simulink model "Vicon_16Aug2012"  (Simulink 7.7)
settings: Solver=ode4  StartTime=0.0  StopTime=inf  FixedStep=sample_time  RelTol=1e-3
InitFcn:
  | sample_time=0.02;
undefined symbols (not defined in the file or in its folder): DiscIntNeverNeededParam
libraries: simulink x7, utility x1
(part 1 of 2)
settings Model: Creator=ttcl3  LastModifiedBy=Zhao Weihua
settings SolverCC: MaxConsecutiveMinStep=auto
settings DebuggingCC: MultiTaskRateTransMsg=warning

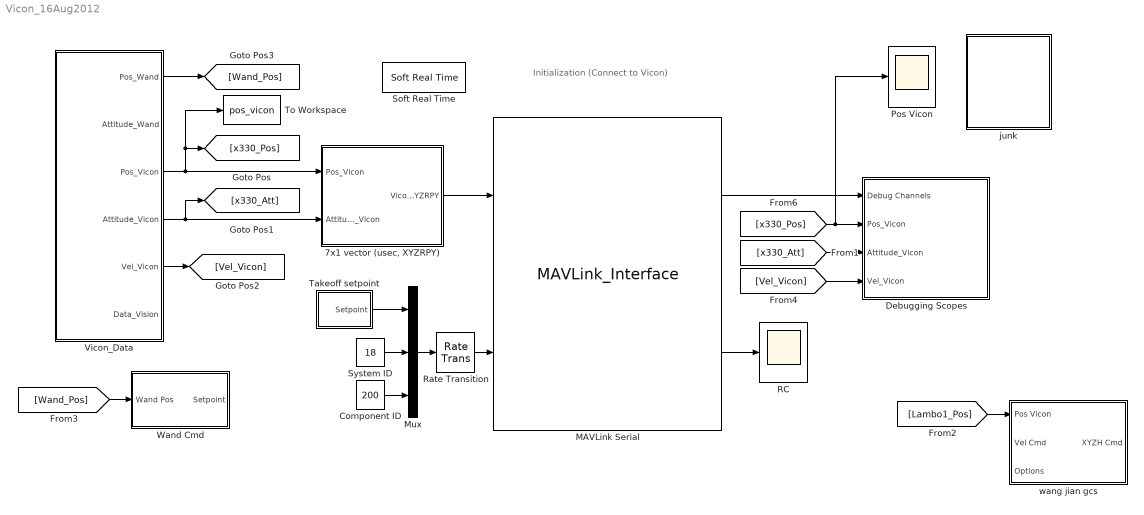
== system Vicon_16Aug2012 ==
  note: Initialization
      | (Connect to Vicon)
  "7x1 vector (usec, XYZRPY)" : Subsystem
  Component ID : Constant  Value=200  SampleTime=sample_time
  Debugging Scopes : Subsystem
  MAVLink Serial : S-Function  FunctionName=MAVLink_Interface  Parameters=COM_Port,Baud_Rate,MSG_INPUT,MSG_OUTPUT  EnableBusSupport=off  mask{COM_Port='COM8', Baud_Rate=57600, HEART_BEAT=off, ATTITUDE_OUT=on, RAW_IMU=off, POSITION_OUT=off, VFR_HUD=off, RC_SCALED=on, SERVO_OUT_RAW=off, VICON_XYZ_RPY_Output=off, SET_MODE=off, DATA_STREAM=off, ATTITUDE_COMMAND=off, ATTITUDE_IN=off, GPS_RAW_IN=off, VFR_HUD_IN=off, VICON_XYZ_RPY=on, VICON_VEL=off, POSITION_DESIRED=on}
      mask prompts: COM_Port "COM Port"; Baud_Rate "Baud Rate"; HEART_BEAT "HEART BEAT"; ATTITUDE_OUT "ATTITUDE"; RAW_IMU "RAW IMU"; POSITION_OUT "GLOBAL POSITION"; VFR_HUD "VFR HUD"; RC_SCALED "RC CHANNELS SCALED"; SERVO_OUT_RAW "SERVO OUTPUT RAW"; VICON_XYZ_RPY_Output "VICON Output"; SET_MODE "SET MODE"; DATA_STREAM "REQUEST DATA STREAM"; ATTITUDE_COMMAND "ATTITUDE COMMAND"; ATTITUDE_IN "ATTITUDE (HIL)"; GPS_RAW_IN "GPS RAW (HIL)"; VFR_HUD_IN "AIRSPEED (HIL)"; VICON_XYZ_RPY "VICON POSITION"; VICON_VEL "VICON SPEED"; POSITION_DESIRED "Position Desired"
      mask init:
      | MSG_ID_NUM_INPUT = [uint8(11) uint8(66) uint8(59) uint8(30) uint8(32) uint8(73) uint8(104) uint8(103) uint8(50)];
      | MSG_ID_NAME_INPUT = [SET_MODE DATA_STREAM ATTITUDE_COMMAND ATTITUDE_IN GPS_RAW_IN VFR_HUD_IN VICON_XYZ_RPY VICON_VEL POSITION_DESIRED];
      | 
      | MSG_ID_NUM_OUTPUT = [uint8(0) uint8(30) uint8(27) uint8(73) uint8(74) uint8(34) uint8(37) uint8(104)];
      | MSG_ID_NAME_OUTPUT = [HEART_BEAT ATTITUDE_OUT RAW_IMU VFR_HUD POSITION_OUT RC_SCALED SERVO_OUT_RAW VICON_XYZ_RPY_Output];
      | 
      | idx_input = find(MSG_ID_NAME_INPUT);
      | MSG_INPUT = MSG_ID_NUM_INPUT(idx_input);
      | 
      | idx_output = find(MSG_ID_NAME_OUTPUT);
      | MSG_OUTPUT = MSG_ID_NUM_OUTPUT(idx_output);
      mask TabNameString: Setting,Setting,Output Message,Output Message,Output Message,Output Message,Output Message,Output Message,Output Message,Output Message,Input Message,Input Message,Input Message,Input Message,Input Message,Input Message,Input Message,Input Message,Input Message
      mask Display:
      | %Label block
      | fprintf('MAVLink Serial\n%s\n%dbps', COM_Port,  Baud_Rate)
      | 
      | %Label input ports
      | 
      | in = 1;
      | if (SET_MODE == 1)
      |     port_label('input', in, 'SET MODE');
      |     in = in + 1;
      | end
      | if (DATA_STREAM == 1)
      |     port_label('input', in, 'REQUEST DATA STREAM');
      |     in = in + 1;
      | end
      | if (ATTITUDE_COMMAND == 1)
      |     port_label('input', in, 'ATTITUDE COMMAND');
      |     in = in + 1;
      | end
      | if (ATTITUDE_IN == 1)
      |     port_label('input', in, 'ATTITUDE (HIL)');
      |     in = in + 1;
      | end
      | if (GPS_RAW_IN == 1)
      |     port_label('input', in, 'GPS RAW (HIL)');
      |     in = in + 1;
      | end
      | if (VFR_HUD_IN == 1)
      |     port_label('input', in, 'AIRSPEED (HIL)');
      |     in = in + 1;
      | end
      | if (VICON_XYZ_RPY == 1)
      |     port_label('input', in, 'VICON XYZ RPY');
      |     in = in + 1;
      | end
      | if (VICON_VEL == 1)
      |     port_label('input', in, 'VICON_VEL');
      |     in = in + 1;
      | end
      | 
      | if (POSITION_DESIRED == 1)
      |     port_label('input', in, 'POSITION_DESIRED');
      |     in = in + 1;
      | end
      | 
      | %Label output ports
      | 
      | out = 1;
      | if (HEART_BEAT == 1)
      |     port_label('output', out, 'HEART BEAT');
      |     out = out + 1;
      | end
      | if (ATTITUDE_OUT == 1)
      |     port_label('output', out, 'ATTITUDE');
      |     out = out + 1;
      | end
      | if (RAW_IMU == 1)
      |     port_label('output', out, 'RAW IMU');
      |     out = out + 1;
      | end
      | if (POSITION_OUT == 1)
      |     port_label('output', out, 'GLOBAL POSITION');
      |     out = out + 1;
      | end
      | if (VFR_HUD == 1)
      |     port_label('output', out, 'VFR HUD');
      |     out = out + 1;
      | end
      | if (RC_SCALED == 1)
      |     port_label('output', out, 'RC CHANNELS SCALED');
      |     out = out + 1;
      | end
      | if (SERVO_OUT_RAW == 1)
      |     port_label('output', out, 'SERVO OUTPUT RAW');
      |     out = out + 1;
      | end
      | % weihua, vicon output
      | if (VICON_XYZ_RPY_Output == 1)
      |     port_label('output', out, 'VICON_XYZ_RPY');
      |     out = out + 1;
      | end
  Mux : Mux  Inputs=3
  Pos Vicon : Scope
      settings: TickLabels=on  TimeRange=30  YMin=-1.5  YMax=0.6  SaveName=ScopeData3  SampleInput=on
  RC : Scope
      settings: TickLabels=on  TimeRange=30  YMin=-1.1  YMax=1.1  SaveName=ScopeData2  SampleInput=on
  Rate Transition : RateTransition  OutPortSampleTime=0.2
  Soft Real Time : utility/Soft Real Time  x=0.8
  System ID : Constant  Value=18  SampleTime=sample_time
  Takeoff setpoint : Subsystem
  To Workspace : ToWorkspace  VariableName=pos_vicon  SampleTime=-1  SaveFormat=Structure
  Vicon_Data : Subsystem
  Wand Cmd : Subsystem
  junk : Subsystem
  wang jian gcs : Subsystem
  wires:
  MAVLink Serial/1 -> Debugging Scopes/1(Debug Channels)
  [x330_Pos] -> Debugging Scopes/2(Pos_Vicon), Pos Vicon/1
  [x330_Att] -> Debugging Scopes/3(Attitude_Vicon)
  "7x1 vector (usec, XYZRPY)"/1(Vicon XYZRPY) -> MAVLink Serial/1
  Vicon_Data/4(Attitude_Vicon) -> [x330_Att], "7x1 vector (usec, XYZRPY)"/2(Attitude_Vicon)
  Mux/1 -> Rate Transition/1
  System ID/1 -> Mux/2
  Component ID/1 -> Mux/3
  [Vel_Vicon] -> Debugging Scopes/4(Vel_Vicon)
  [Lambo1_Pos] -> wang jian gcs/1(Pos Vicon)
  Vicon_Data/5(Vel_Vicon) -> [Vel_Vicon]
  Vicon_Data/3(Pos_Vicon) -> "7x1 vector (usec, XYZRPY)"/1(Pos_Vicon), [x330_Pos], To Workspace/1
  [Wand_Pos] -> Wand Cmd/1(Wand Pos)
  Vicon_Data/1(Pos_Wand) -> [Wand_Pos]
  MAVLink Serial/2 -> RC/1
  Takeoff setpoint/1(Setpoint) -> Mux/1
  Rate Transition/1 -> MAVLink Serial/2

== system Vicon_16Aug2012/7x1 vector (usec, XYZRPY) ==
  Pos_Vicon : Inport
  Attitude_Vicon : Inport  Port=2
  Mux1 : Mux  Inputs=3
  usec : Constant  Value=0
  Vicon XYZRPY : Outport
  wires:
  usec/1 -> Mux1/1
  Pos_Vicon/1 -> Mux1/2
  Attitude_Vicon/1 -> Mux1/3
  Mux1/1 -> Vicon XYZRPY/1

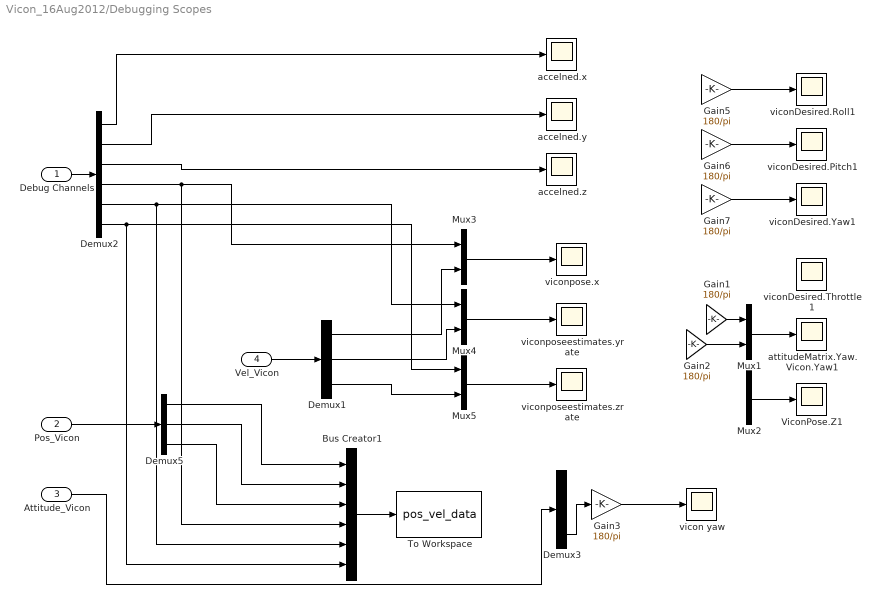
== system Vicon_16Aug2012/Debugging Scopes ==
  Debug Channels : Inport
  Pos_Vicon : Inport  Port=2
  Attitude_Vicon : Inport  Port=3
  Vel_Vicon : Inport  Port=4
  Bus Creator1 : BusCreator  Inputs=6
  Demux1 : Demux  Outputs=3
  Demux2 : Demux  Outputs=6
  Demux3 : Demux  Outputs=3
  Demux5 : Demux  Outputs=3
  Gain{1..3,5..7} (6 alike) : Gain  Gain=180/pi
  Mux{1..5} (5 alike) : Mux  Inputs=2
  To Workspace : ToWorkspace  VariableName=pos_vel_data  SampleTime=sample_time  SaveFormat=Structure With Time
  ViconPose.Z1 : Scope
      settings: TickLabels=on  TimeRange=60  YMin=-0.475  YMax=-0.2  SaveName=ScopeData9  SampleInput=on
  accelned.x : Scope
      settings: TickLabels=on  TimeRange=60  YMin=-0.06  YMax=-0.0325  SampleInput=on
  accelned.y : Scope
      settings: TickLabels=on  TimeRange=25  YMin=4.12  YMax=4.34  SaveName=ScopeData13  SampleInput=on
  accelned.z : Scope
      settings: TickLabels=on  TimeRange=60  YMin=0.18  YMax=0.31  SaveName=ScopeData14  SampleInput=on
  attitudeMatrix.Yaw. Vicon.Yaw1 : Scope
      settings: TickLabels=on  TimeRange=60  YMin=-81  YMax=-72.5  SaveName=ScopeData15  SampleInput=on
  vicon yaw : Scope
      settings: TickLabels=on  TimeRange=60  YMin=-180  YMax=180  SaveName=ScopeData17  SampleInput=on
  viconDesired.Pitch1 : Scope
      settings: TickLabels=on  TimeRange=25  YMin=-10.5  YMax=1  SaveName=ScopeData6  SampleInput=on
  viconDesired.Roll1 : Scope
      settings: TickLabels=on  TimeRange=60  YMax=7  SaveName=ScopeData7  SampleInput=on
  viconDesired.Throttle1 : Scope
      settings: TickLabels=on  TimeRange=60  YMin=0  YMax=0.5  SaveName=ScopeData16  SampleInput=on
  viconDesired.Yaw1 : Scope
      settings: TickLabels=on  TimeRange=60  YMin=-0.125  YMax=-0.0725  SaveName=ScopeData8  SampleInput=on
  viconpose.x : Scope
      settings: TickLabels=on  TimeRange=60  YMin=-4.75  YMax=0.5  SampleInput=on
  viconposeestimates.yrate : Scope
      settings: TickLabels=on  TimeRange=99.52455918402114  YMin=-0.5  YMax=4.25  SaveName=ScopeData11  SampleInput=on
  viconposeestimates.zrate : Scope
      settings: TickLabels=on  TimeRange=60  YMin=-0.25  YMax=2.75  SaveName=ScopeData12  SampleInput=on
  wires:
  Demux2/1 -> accelned.x/1
  Demux2/2 -> accelned.y/1
  Demux2/3 -> accelned.z/1
  Demux5/3 -> Bus Creator1/3
  Demux5/1 -> Bus Creator1/1
  Demux5/2 -> Bus Creator1/2
  Bus Creator1/1 -> To Workspace/1
  Debug Channels/1 -> Demux2/1
  Pos_Vicon/1 -> Demux5/1
  Gain5/1 -> viconDesired.Roll1/1
  Gain6/1 -> viconDesired.Pitch1/1
  Gain7/1 -> viconDesired.Yaw1/1
  Mux1/1 -> attitudeMatrix.Yaw. Vicon.Yaw1/1
  Mux2/1 -> ViconPose.Z1/1
  Gain1/1 -> Mux1/1
  Gain2/1 -> Mux1/2
  Vel_Vicon/1 -> Demux1/1
  Demux2/4 -> Mux3/1, Bus Creator1/4
  Demux2/5 -> Mux4/1, Bus Creator1/5
  Demux2/6 -> Mux5/1, Bus Creator1/6
  Mux3/1 -> viconpose.x/1
  Mux4/1 -> viconposeestimates.yrate/1
  Mux5/1 -> viconposeestimates.zrate/1
  Gain3/1 -> vicon yaw/1
  Demux3/3 -> Gain3/1
  Attitude_Vicon/1 -> Demux3/1
  Demux1/1 -> Mux3/2
  Demux1/2 -> Mux4/2
  Demux1/3 -> Mux5/2

== system Vicon_16Aug2012/Takeoff setpoint ==
  Des_X : Constant  Value=0  SampleTime=sample_time
  Des_Y : Constant  Value=0  SampleTime=sample_time
  Des_Yaw : Constant  Value=0  SampleTime=sample_time
  Des_Z : Constant  Value=-0.8  SampleTime=sample_time
  Mux3 : Mux
  Setpoint : Outport
  wires:
  Des_X/1 -> Mux3/1
  Des_Y/1 -> Mux3/2
  Des_Z/1 -> Mux3/3
  Des_Yaw/1 -> Mux3/4
  Mux3/1 -> Setpoint/1

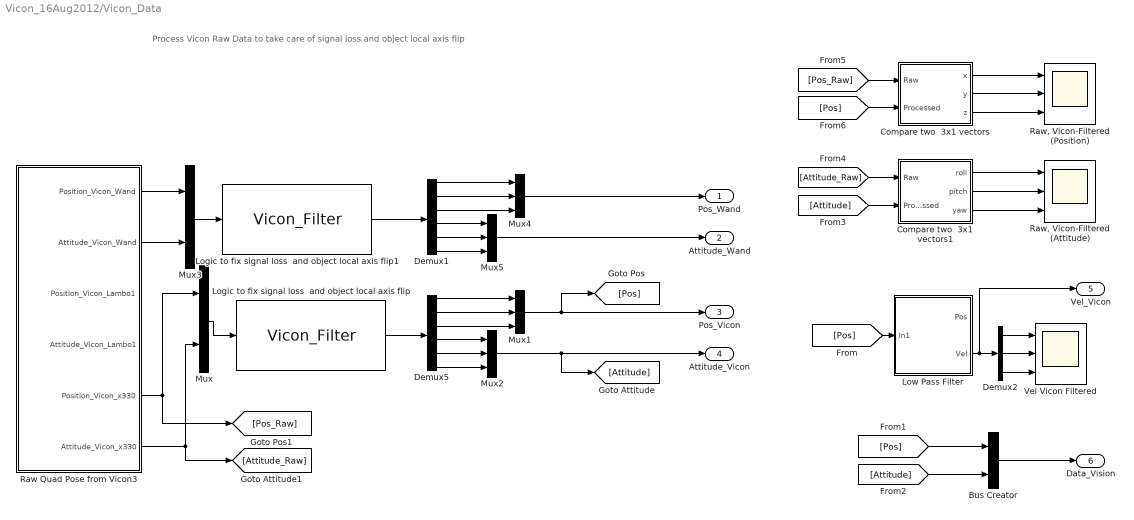
== system Vicon_16Aug2012/Vicon_Data ==
  note: Process Vicon Raw Data to take care of signal loss and object local axis flip
  Bus Creator : BusCreator  Inputs=2
  Compare two  3x1 vectors : Subsystem
  Compare two  3x1 vectors1 : Subsystem
  Demux1 : Demux  Outputs=6
  Demux2 : Demux  Outputs=3
  Demux5 : Demux  Outputs=6
  Logic to fix signal loss  and object local axis flip : M-S-Function  FunctionName=Vicon_Filter
  Logic to fix signal loss  and object local axis flip1 : M-S-Function  FunctionName=Vicon_Filter
  Low Pass Filter : Subsystem
  Mux : Mux  Inputs=2
  Mux{1..2,4..5} (4 alike) : Mux  Inputs=3
  Mux3 : Mux  Inputs=2
  Raw Quad Pose from Vicon3 : Subsystem
  "Raw, Vicon-Filtered (Attitude)" : Scope  NumInputPorts=3
      settings: TimeRange=50  YMin=-3.14159~-1~-3.5  YMax=3.14159~1~3.5  SaveName=ScopeData4
  "Raw, Vicon-Filtered (Position)" : Scope  NumInputPorts=3
      settings: TimeRange=50  YMin=-2.09~2.281~-0.0655  YMax=-2.055~2.293~-0.063  SaveName=ScopeData10
  "Vel Vicon Filtered " : Scope  NumInputPorts=3
      settings: YMin=-0.7~-1~-9  YMax=0.4~7.5~0.5  SaveName=ScopeData5
  Pos_Wand : Outport
  Attitude_Wand : Outport  Port=2
  Pos_Vicon : Outport  Port=3
  Attitude_Vicon : Outport  Port=4
  Vel_Vicon : Outport  Port=5
  Data_Vision : Outport  Port=6
  wires:
  Demux2/1 -> "Vel Vicon Filtered "/1
  Demux2/2 -> "Vel Vicon Filtered "/2
  Demux2/3 -> "Vel Vicon Filtered "/3
  Compare two  3x1 vectors/1(x) -> "Raw, Vicon-Filtered (Position)"/1
  Compare two  3x1 vectors/2(y) -> "Raw, Vicon-Filtered (Position)"/2
  Low Pass Filter/2(Vel) -> Demux2/1, Vel_Vicon/1
  Mux/1 -> Logic to fix signal loss  and object local axis flip/1
  Logic to fix signal loss  and object local axis flip/1 -> Demux5/1
  Demux5/1 -> Mux1/1
  Demux5/2 -> Mux1/2
  Demux5/3 -> Mux1/3
  Demux5/4 -> Mux2/1
  Demux5/5 -> Mux2/2
  Demux5/6 -> Mux2/3
  Mux2/1 -> Attitude_Vicon/1, [Attitude]
  [Pos] -> Low Pass Filter/1(In1)
  Compare two  3x1 vectors/3(z) -> "Raw, Vicon-Filtered (Position)"/3
  Compare two  3x1 vectors1/1(roll) -> "Raw, Vicon-Filtered (Attitude)"/1
  Compare two  3x1 vectors1/2(pitch) -> "Raw, Vicon-Filtered (Attitude)"/2
  Mux1/1 -> Pos_Vicon/1, [Pos]
  Compare two  3x1 vectors1/3(yaw) -> "Raw, Vicon-Filtered (Attitude)"/3
  [Attitude_Raw] -> Compare two  3x1 vectors1/1(Raw)
  [Attitude] -> Compare two  3x1 vectors1/2(Processed)
  [Pos_Raw] -> Compare two  3x1 vectors/1(Raw)
  [Pos] -> Compare two  3x1 vectors/2(Processed)
  [Pos] -> Bus Creator/1
  [Attitude] -> Bus Creator/2
  Bus Creator/1 -> Data_Vision/1
  Mux3/1 -> Logic to fix signal loss  and object local axis flip1/1
  Logic to fix signal loss  and object local axis flip1/1 -> Demux1/1
  Demux1/1 -> Mux4/1
  Demux1/2 -> Mux4/2
  Demux1/3 -> Mux4/3
  Demux1/4 -> Mux5/1
  Demux1/5 -> Mux5/2
  Demux1/6 -> Mux5/3
  Mux5/1 -> Attitude_Wand/1
  Mux4/1 -> Pos_Wand/1
  Raw Quad Pose from Vicon3/1(Position_Vicon_Wand) -> Mux3/1
  Raw Quad Pose from Vicon3/2(Attitude_Vicon_Wand) -> Mux3/2
  Raw Quad Pose from Vicon3/5(Position_Vicon_x330) -> Mux/1, [Pos_Raw]
  Raw Quad Pose from Vicon3/6(Attitude_Vicon_x330) -> Mux/2, [Attitude_Raw]

== system Vicon_16Aug2012/Wand Cmd ==
  Wand Pos : Inport
  Add : Sum
  Add1 : Sum
  Add2 : Sum
  Demux : Demux  Outputs=3
  Des_Yaw : Constant  Value=0  SampleTime=sample_time
  Height 1m (testing) : Constant  Value=-1  SampleTime=sample_time
  Mux1 : Mux
  X offset : Constant  Value=-0.5
  Y offset : Constant  Value=-0.5
  Z offset : Constant  Value=-0.5
  Setpoint : Outport
  wires:
  Wand Pos/1 -> Demux/1
  Mux1/1 -> Setpoint/1
  Demux/1 -> Add/1
  X offset/1 -> Add/2
  Demux/2 -> Add1/1
  Y offset/1 -> Add1/2
  Demux/3 -> Add2/1
  Z offset/1 -> Add2/2
  Add/1 -> Mux1/1
  Add1/1 -> Mux1/2
  Des_Yaw/1 -> Mux1/4
  Height 1m (testing)/1 -> Mux1/3

== system Vicon_16Aug2012/junk ==
  note: 2 Take off
      | 5 Step (setpoint)
      | 6 Land
  4x1 vector : Subsystem
  4x1 vector (usec; vel)1 : Subsystem
  7x1 vector : Subsystem
  Autonomous Takeoff and Position Hold1 : M-S-Function  FunctionName=Last_Position_Hold
      mask Display:
      | port_label('output', 1, 'Processed Setpoint')
      | 
      | port_label('input', 1, 'Desired Setpoint')
      | 
      | port_label('input', 2, 'Vicon Pose')
      | 
      | port_label('input', 3, 'Vicon Attitude')
      | 
      | port_label('input', 4, 'RC Channel 5')
  Constant3 : Constant  Value=2
  Constant4 : Constant  Value=6
  XYZY : Subsystem

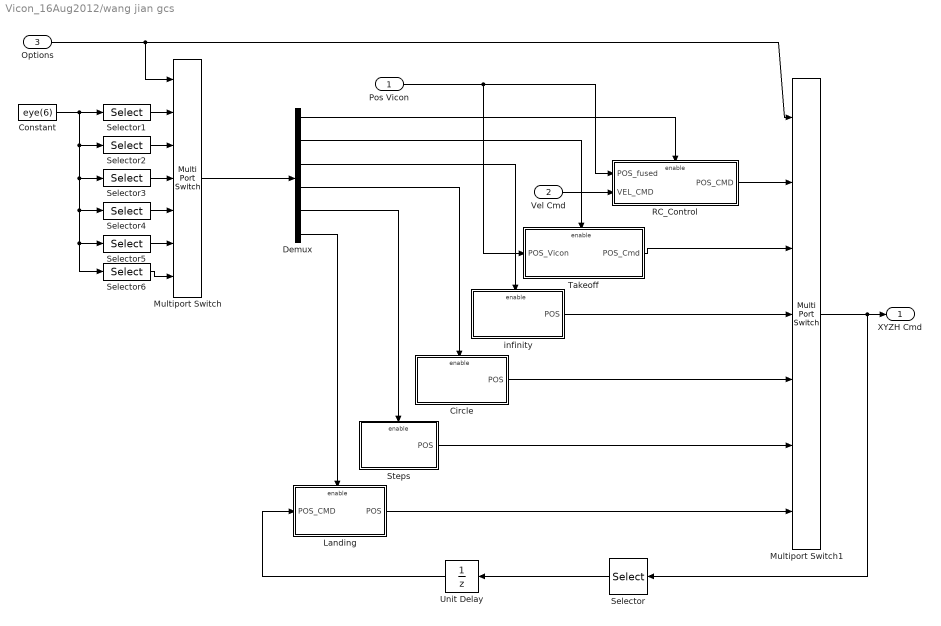
== system Vicon_16Aug2012/wang jian gcs ==
  Pos Vicon : Inport
  Vel Cmd : Inport  Port=2
  Options : Inport  Port=3
  Circle : Subsystem
  Constant : Constant  Value=eye(6)
  Demux : Demux  Outputs=6
  Landing : Subsystem
  Multiport Switch : MultiPortSwitch  Inputs=6  DiagnosticForDefault=Warning  zeroidx=off
  Multiport Switch1 : MultiPortSwitch  Inputs=6  DiagnosticForDefault=Warning  zeroidx=off
  RC_Control : Subsystem
  Selector : Selector  InputPortWidth=4  IndexOptions=Index vector (dialog)  Indices=[1 2 3]  OutputSizes=1
  Selector1 : Selector  NumberOfDimensions=2  InputPortWidth=3  IndexOptions=Select all,Index vector (dialog)  Indices=1,1  OutputSizes=1,1
  Selector2 : Selector  NumberOfDimensions=2  InputPortWidth=3  IndexOptions=Select all,Index vector (dialog)  Indices=1,2  OutputSizes=1,1
  Selector3 : Selector  NumberOfDimensions=2  InputPortWidth=3  IndexOptions=Select all,Index vector (dialog)  Indices=1,3  OutputSizes=1,1
  Selector4 : Selector  NumberOfDimensions=2  InputPortWidth=3  IndexOptions=Select all,Index vector (dialog)  Indices=1,4  OutputSizes=1,1
  Selector5 : Selector  NumberOfDimensions=2  InputPortWidth=3  IndexOptions=Select all,Index vector (dialog)  Indices=1,5  OutputSizes=1,1
  Selector6 : Selector  NumberOfDimensions=2  InputPortWidth=3  IndexOptions=Select all,Index vector (dialog)  Indices=1,6  OutputSizes=1,1
  Steps : Subsystem
  Takeoff : Subsystem
  Unit Delay : UnitDelay  SampleTime=-1
  infinity : Subsystem
  XYZH Cmd : Outport
  wires:
  Options/1 -> Multiport Switch1/1, Multiport Switch/1
  Vel Cmd/1 -> RC_Control/2(VEL_CMD)
  Selector/1 -> Unit Delay/1
  RC_Control/1(POS_CMD) -> Multiport Switch1/2
  Unit Delay/1 -> Landing/1(POS_CMD)
  Pos Vicon/1 -> Takeoff/1(POS_Vicon), RC_Control/1(POS_fused)
  Demux/4 -> Circle/Enable
  Demux/3 -> infinity/Enable
  Demux/2 -> Takeoff/Enable
  Demux/1 -> RC_Control/Enable
  Circle/1(POS) -> Multiport Switch1/5
  infinity/1(POS) -> Multiport Switch1/4
  Multiport Switch1/1 -> XYZH Cmd/1, Selector/1
  Multiport Switch/1 -> Demux/1
  Constant/1 -> Selector2/1, Selector1/1, Selector3/1, Selector4/1, Selector5/1, Selector6/1
  Selector1/1 -> Multiport Switch/2
  Selector2/1 -> Multiport Switch/3
  Selector3/1 -> Multiport Switch/4
  Selector4/1 -> Multiport Switch/5
  Selector5/1 -> Multiport Switch/6
  Selector6/1 -> Multiport Switch/7
  Demux/5 -> Steps/Enable
  Demux/6 -> Landing/Enable
  Steps/1(POS) -> Multiport Switch1/6
  Landing/1(POS) -> Multiport Switch1/7
  Takeoff/1(POS_Cmd) -> Multiport Switch1/3

== system Vicon_16Aug2012/Vicon_Data/Compare two  3x1 vectors ==
  Raw : Inport
  Processed : Inport  Port=2
  Demux6 : Demux  Outputs=3
  Demux7 : Demux  Outputs=3
  Mux : Mux  Inputs=2
  Mux1 : Mux  Inputs=2
  Mux2 : Mux  Inputs=2
  x : Outport
  y : Outport  Port=2
  z : Outport  Port=3
  wires:
  Demux6/1 -> Mux/1
  Demux6/2 -> Mux1/1
  Demux7/2 -> Mux1/2
  Demux6/3 -> Mux2/1
  Demux7/3 -> Mux2/2
  Raw/1 -> Demux6/1
  Processed/1 -> Demux7/1
  Mux/1 -> x/1
  Mux1/1 -> y/1
  Mux2/1 -> z/1
  Demux7/1 -> Mux/2

== system Vicon_16Aug2012/Vicon_Data/Compare two  3x1 vectors1 ==
  Raw : Inport
  Processed : Inport  Port=2
  Demux6 : Demux  Outputs=3
  Demux7 : Demux  Outputs=3
  Mux : Mux  Inputs=2
  Mux1 : Mux  Inputs=2
  Mux2 : Mux  Inputs=2
  roll : Outport
  pitch : Outport  Port=2
  yaw : Outport  Port=3
  wires:
  Demux7/1 -> Mux/2
  Mux2/1 -> yaw/1
  Mux1/1 -> pitch/1
  Mux/1 -> roll/1
  Processed/1 -> Demux7/1
  Raw/1 -> Demux6/1
  Demux7/3 -> Mux2/2
  Demux6/3 -> Mux2/1
  Demux7/2 -> Mux1/2
  Demux6/2 -> Mux1/1
  Demux6/1 -> Mux/1

== system Vicon_16Aug2012/Vicon_Data/Low Pass Filter ==
  In1 : Inport
  Gain : Gain  Gain=3
  Integrator : Integrator
  Sum : Sum  Inputs=|+-
  Pos : Outport
  Vel : Outport  Port=2
  wires:
  Sum/1 -> Gain/1
  Gain/1 -> Integrator/1, Vel/1
  Integrator/1 -> Pos/1, Sum/2
  In1/1 -> Sum/1

== system Vicon_16Aug2012/Vicon_Data/Raw Quad Pose from Vicon3 ==
  Constant : Constant
  Demux : Demux  Outputs=3
  Interpreted MATLAB Function : MATLABFcn  MATLABFcn=GetViconPose
  Process Vicon Raw Data : Subsystem
  Process Vicon Raw Data1 : Subsystem
  Process Vicon Raw Data2 : Subsystem
  Position_Vicon_Wand : Outport
  Attitude_Vicon_Wand : Outport  Port=2
  Position_Vicon_Lambo1 : Outport  Port=3
  Attitude_Vicon_Lambo1 : Outport  Port=4
  Position_Vicon_x330 : Outport  Port=5
  Attitude_Vicon_x330 : Outport  Port=6
  wires:
  Process Vicon Raw Data/2(Attitude) -> Attitude_Vicon_Wand/1
  Process Vicon Raw Data/1(Position) -> Position_Vicon_Wand/1
  Process Vicon Raw Data1/2(Attitude) -> Attitude_Vicon_Lambo1/1
  Process Vicon Raw Data1/1(Position) -> Position_Vicon_Lambo1/1
  Process Vicon Raw Data2/2(Attitude) -> Attitude_Vicon_x330/1
  Process Vicon Raw Data2/1(Position) -> Position_Vicon_x330/1
  Constant/1 -> Interpreted MATLAB Function/1
  Interpreted MATLAB Function/1 -> Demux/1
  Demux/1 -> Process Vicon Raw Data/1(Vicon Raw)
  Demux/2 -> Process Vicon Raw Data1/1(Vicon Raw)
  Demux/3 -> Process Vicon Raw Data2/1(Vicon Raw)

== system Vicon_16Aug2012/junk/4x1 vector ==
  Mux2 : Mux
  Vx : Constant  Value=0  SampleTime=0.02
  Vy : Constant  Value=0  SampleTime=0.02
  Vz : Constant  Value=0  SampleTime=0.02
  usec_Speed : Constant  Value=0  SampleTime=0.02
  Debug signals : Outport
  wires:
  usec_Speed/1 -> Mux2/1
  Vx/1 -> Mux2/2
  Vy/1 -> Mux2/3
  Vz/1 -> Mux2/4
  Mux2/1 -> Debug signals/1

== system Vicon_16Aug2012/junk/4x1 vector (usec; vel)1 ==
  In1 : Inport
  Demux6 : Demux  Outputs=3
  Mux2 : Mux
  usec_Speed : Constant  Value=0  SampleTime=0.02
  Vicon velocity : Outport
  wires:
  In1/1 -> Demux6/1
  Mux2/1 -> Vicon velocity/1
  Demux6/3 -> Mux2/4
  Demux6/2 -> Mux2/3
  Demux6/1 -> Mux2/2
  usec_Speed/1 -> Mux2/1

== system Vicon_16Aug2012/junk/7x1 vector ==
  Mux : Mux  Inputs=7
  Pitch : Constant  Value=5
  Pulse Generator1 : DiscretePulseGenerator  PulseType=Time based  Period=6  PulseWidth=50  SampleTime=-1
  Roll : Constant  Value=4
  Sine Wave1 : Sin  SampleTime=sample_time
  Sine Wave2 : Sin  Frequency=0.5  SampleTime=sample_time
  Yaw : Constant  Value=6
  Z : Constant  Value=3
  usec : Constant  Value=0
  Debug signals : Outport
  wires:
  usec/1 -> Mux/1
  Sine Wave2/1 -> Mux/2
  Sine Wave1/1 -> Mux/3
  Z/1 -> Mux/4
  Roll/1 -> Mux/5
  Pitch/1 -> Mux/6
  Yaw/1 -> Mux/7
  Mux/1 -> Debug signals/1

== system Vicon_16Aug2012/junk/XYZY ==
  Des_X : Constant  Value=0  SampleTime=sample_time
  Des_Y : Constant  Value=0  SampleTime=sample_time
  Des_Yaw : Constant  Value=0  SampleTime=sample_time
  Des_Z : Constant  Value=-1  SampleTime=sample_time
  Mux3 : Mux
  Setpoint : Outport
  wires:
  Des_X/1 -> Mux3/1
  Des_Y/1 -> Mux3/2
  Des_Z/1 -> Mux3/3
  Des_Yaw/1 -> Mux3/4
  Mux3/1 -> Setpoint/1

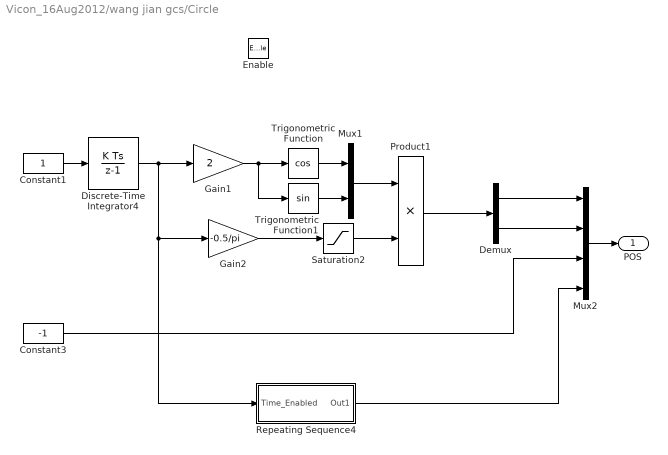
== system Vicon_16Aug2012/wang jian gcs/Circle ==
  Enable : EnablePort  StatesWhenEnabling=reset
  Constant1 : Constant  OutDataTypeStr=double
  Constant3 : Constant  Value=-1  OutDataTypeStr=double
  Demux : Demux  Outputs=2
  Discrete-Time Integrator4 : DiscreteIntegrator  SampleTime=-1  ICPrevOutput=DiscIntNeverNeededParam  ICPrevScaledInput=DiscIntNeverNeededParam
  Gain1 : Gain  Gain=2
  Gain2 : Gain  Gain=-0.5/pi
  Mux1 : Mux  Inputs=2
  Mux2 : Mux
  Product1 : Product  RndMeth=Zero
  Repeating Sequence4 : Subsystem  mask(Repeating table){rep_seq_t=[0 1*pi 1*pi 6*pi 6*pi 7*pi], rep_seq_y=[0 0 -1 -1 0 0]*-2}
      mask prompts: rep_seq_t "Time values:"; rep_seq_y "Output values:"
      mask help: Output a repeating sequence of numbers specified in a table of time-value pairs. Values of time should be monotonically increasing.
      mask init:
      | if (length(rep_seq_t) ~= length(rep_seq_y)),
      |   error('Length of time vector and output vector must be the same.')
      | end
      | dbl_rep_seq_t = double(rep_seq_t);
      | dbl_rep_seq_y = double(rep_seq_y);
      | period = max(dbl_rep_seq_t) - min(dbl_rep_seq_t);
      | period = str2num(sprintf('%0.5g',period));
      | s = round(length(dbl_rep_seq_t)/50);
      | if s > 0
      |   pts = [1:s:length(dbl_rep_seq_t)];
      |   L   = length(pts);
      | else
      |   L   = length(dbl_rep_seq_t);
      |   pts = [1:L];
      | end
      | 
      | disp_seq_t = reshape(dbl_rep_seq_t(pts),L,1);
      | disp_seq_y = reshape(dbl_rep_seq_y(pts),L,1);
      | disp_period = max(disp_seq_t) - min(disp_seq_t);
      | 
      | disp_seq_t  = repmat(disp_seq_t,1,3) + (ones(L,1)*(disp_period*[0,1,2]));
      | disp_seq_t = [ disp_seq_t(:); disp_seq_t(end) ];
      | disp_seq_y = repmat(disp_seq_y,1,3);
      | disp_seq_y = [ disp_seq_y(:); disp_seq_y(1) ];
      mask Help: Repeats cycle given in table. Time values should be monotonically increasing.
      mask Display: plot( disp_seq_t, disp_seq_y )
  Saturation2 : Saturate  UpperLimit=0  LowerLimit=-1.7  RndMeth=Nearest
  Trigonometric Function : Trigonometry  Operator=cos
  Trigonometric Function1 : Trigonometry
  POS : Outport  InitialOutput=[0 0 -0.8 0]
  wires:
  Saturation2/1 -> Product1/2
  Gain2/1 -> Saturation2/1
  Constant3/1 -> Mux2/3
  Discrete-Time Integrator4/1 -> Gain1/1, Gain2/1, Repeating Sequence4/1(Time_Enabled)
  Mux1/1 -> Product1/1
  Trigonometric Function/1 -> Mux1/1
  Trigonometric Function1/1 -> Mux1/2
  Mux2/1 -> POS/1
  Product1/1 -> Demux/1
  Demux/1 -> Mux2/1
  Demux/2 -> Mux2/2
  Gain1/1 -> Trigonometric Function1/1, Trigonometric Function/1
  Constant1/1 -> Discrete-Time Integrator4/1
  Repeating Sequence4/1(Out1) -> Mux2/4

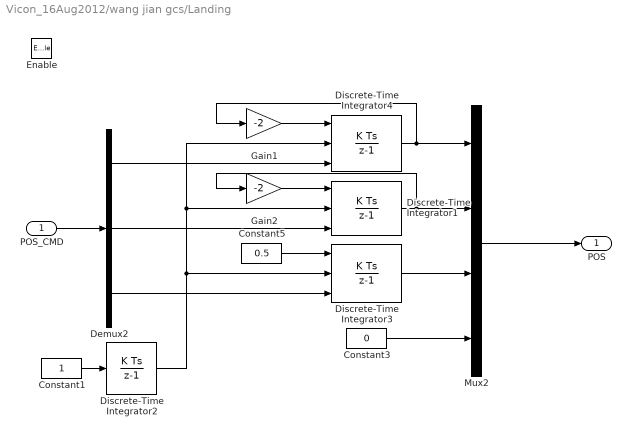
== system Vicon_16Aug2012/wang jian gcs/Landing ==
  POS_CMD : Inport
  Enable : EnablePort  StatesWhenEnabling=reset
  Constant1 : Constant  OutDataTypeStr=double
  Constant3 : Constant  Value=0  OutDataTypeStr=double
  Constant5 : Constant  Value=0.5  OutDataTypeStr=double
  Demux2 : Demux  Outputs=3
  Discrete-Time Integrator1 : DiscreteIntegrator  ExternalReset=rising  InitialConditionSource=external  SampleTime=-1  LimitOutput=on  UpperSaturationLimit=0.8  LowerSaturationLimit=-0.8  ICPrevOutput=DiscIntNeverNeededParam  ICPrevScaledInput=DiscIntNeverNeededParam
  Discrete-Time Integrator2 : DiscreteIntegrator  SampleTime=-1  ICPrevOutput=DiscIntNeverNeededParam  ICPrevScaledInput=DiscIntNeverNeededParam
  Discrete-Time Integrator3 : DiscreteIntegrator  ExternalReset=either  InitialConditionSource=external  SampleTime=-1  LimitOutput=on  UpperSaturationLimit=0.2  LowerSaturationLimit=-1.8  ICPrevOutput=DiscIntNeverNeededParam  ICPrevScaledInput=DiscIntNeverNeededParam
  Discrete-Time Integrator4 : DiscreteIntegrator  ExternalReset=rising  InitialConditionSource=external  SampleTime=-1  LimitOutput=on  UpperSaturationLimit=0.5  LowerSaturationLimit=-0.5  ICPrevOutput=DiscIntNeverNeededParam  ICPrevScaledInput=DiscIntNeverNeededParam
  Gain1 : Gain  Gain=-2
  Gain2 : Gain  Gain=-2
  Mux2 : Mux
  POS : Outport  InitialOutput=[0 0 0 0]
  wires:
  Constant5/1 -> Discrete-Time Integrator3/1
  Mux2/1 -> POS/1
  Constant3/1 -> Mux2/4
  Constant1/1 -> Discrete-Time Integrator2/1
  Discrete-Time Integrator2/1 -> Discrete-Time Integrator3/2, Discrete-Time Integrator1/2, Discrete-Time Integrator4/2
  Discrete-Time Integrator3/1 -> Mux2/3
  Discrete-Time Integrator4/1 -> Mux2/1, Gain1/1
  Discrete-Time Integrator1/1 -> Mux2/2, Gain2/1
  POS_CMD/1 -> Demux2/1
  Demux2/1 -> Discrete-Time Integrator4/3
  Demux2/2 -> Discrete-Time Integrator1/3
  Demux2/3 -> Discrete-Time Integrator3/3
  Gain1/1 -> Discrete-Time Integrator4/1
  Gain2/1 -> Discrete-Time Integrator1/1

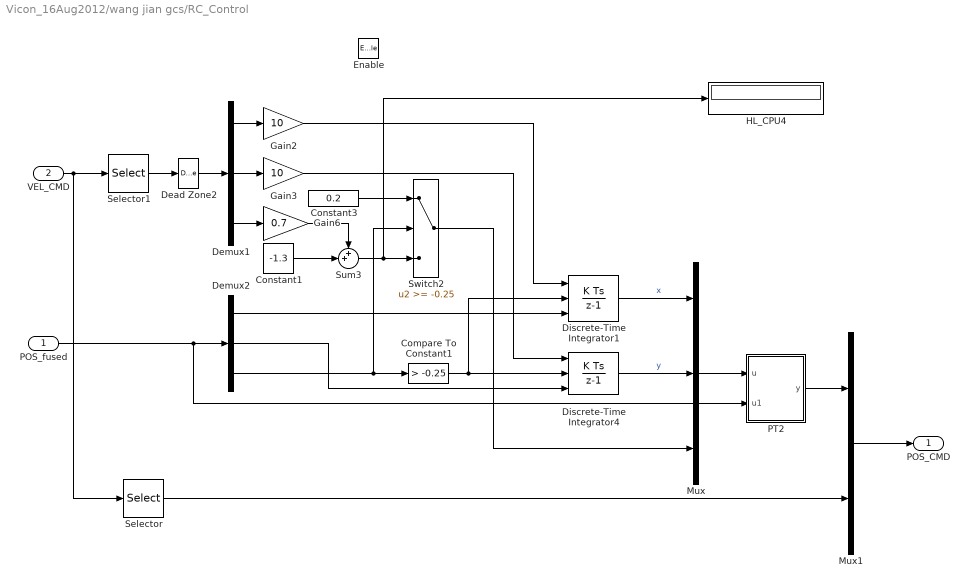
== system Vicon_16Aug2012/wang jian gcs/RC_Control ==
  POS_fused : Inport
  VEL_CMD : Inport  Port=2
  Enable : EnablePort  StatesWhenEnabling=reset
  Compare To Constant1 : simulink/Logic and Bit Operations/Compare To Constant  SystemSampleTime=-1  relop=>  const=-0.25  LogicOutDataTypeMode=uint8
  Constant1 : Constant  Value=-1.3
  Constant3 : Constant  Value=0.2  VectorParams1D=off  OutDataTypeStr=double
  Dead Zone2 : DeadZone  LowerValue=-0.1  UpperValue=0.1  SaturateOnIntegerOverflow=on
  Demux1 : Demux  Outputs=3
  Demux2 : Demux  Outputs=3
  Discrete-Time Integrator1 : DiscreteIntegrator  ExternalReset=level  InitialConditionSource=external  SampleTime=sample_time  LimitOutput=on  UpperSaturationLimit=1.5  LowerSaturationLimit=-1.5  ICPrevOutput=DiscIntNeverNeededParam  ICPrevScaledInput=DiscIntNeverNeededParam
  Discrete-Time Integrator4 : DiscreteIntegrator  ExternalReset=level  InitialConditionSource=external  SampleTime=sample_time  LimitOutput=on  UpperSaturationLimit=3  LowerSaturationLimit=-4  ICPrevOutput=DiscIntNeverNeededParam  ICPrevScaledInput=DiscIntNeverNeededParam
  Gain2 : Gain  Gain=10  ParamDataTypeStr=double  OutDataTypeStr=double
  Gain3 : Gain  Gain=10  ParamDataTypeStr=double  OutDataTypeStr=double
  Gain6 : Gain  Gain=0.7
  HL_CPU4 : Display
  Mux : Mux  Inputs=3
  Mux1 : Mux  Inputs=2
  PT2 : Subsystem  mask(First Order Lag Element){T=0.1}
      mask help:
      | First order lag element with external reset flag (rising edge)
      | and external initial condition.
      mask Help:
      | First order lag element with external reset flag (rising edge)
      | and external initial condition.
      mask Display: disp('LP')
  Selector : Selector  InputPortWidth=4  IndexOptions=Index vector (dialog)  Indices=4  OutputSizes=1
  Selector1 : Selector  InputPortWidth=4  IndexOptions=Index vector (dialog)  Indices=1:3  OutputSizes=1
  Sum3 : Sum  Inputs=++|
  Switch2 : Switch  Threshold=-0.25
  POS_CMD : Outport  InitialOutput=[0 0 0.2 0]
  wires:
  Selector1/1 -> Dead Zone2/1
  Selector/1 -> Mux1/2
  Compare To Constant1/1 -> Discrete-Time Integrator1/2, Discrete-Time Integrator4/2
  Demux2/2 -> Discrete-Time Integrator4/3
  Demux2/1 -> Discrete-Time Integrator1/3
  Demux2/3 -> Compare To Constant1/1, Switch2/2
  POS_fused/1 -> Demux2/1, PT2/2(u1)
  Discrete-Time Integrator1/1 -> Mux/1  "x"
  Discrete-Time Integrator4/1 -> Mux/2  "y"
  Mux/1 -> PT2/1(u)
  Demux1/3 -> Gain6/1
  Dead Zone2/1 -> Demux1/1
  VEL_CMD/1 -> Selector1/1, Selector/1
  Demux1/1 -> Gain2/1
  Demux1/2 -> Gain3/1
  Gain2/1 -> Discrete-Time Integrator1/1
  Gain3/1 -> Discrete-Time Integrator4/1
  Gain6/1 -> Sum3/1
  Constant1/1 -> Sum3/2
  Sum3/1 -> HL_CPU4/1, Switch2/3
  Constant3/1 -> Switch2/1
  Switch2/1 -> Mux/3
  PT2/1(y) -> Mux1/1
  Mux1/1 -> POS_CMD/1

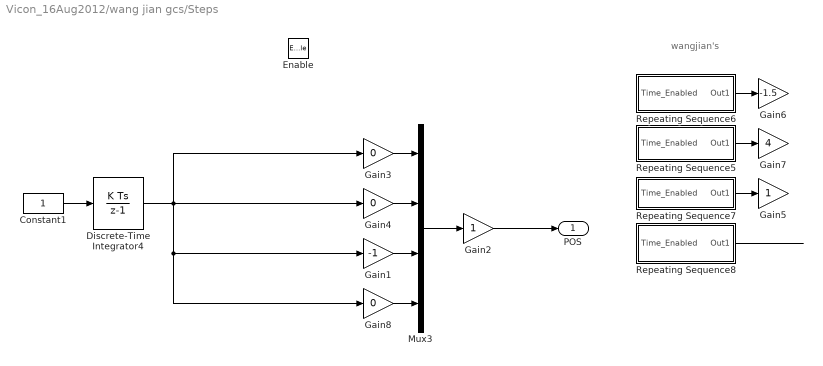
== system Vicon_16Aug2012/wang jian gcs/Steps ==
  note: wangjian's
  Enable : EnablePort  StatesWhenEnabling=reset
  Constant1 : Constant  OutDataTypeStr=double
  Discrete-Time Integrator4 : DiscreteIntegrator  SampleTime=-1  ICPrevOutput=DiscIntNeverNeededParam  ICPrevScaledInput=DiscIntNeverNeededParam
  Gain1 : Gain  Gain=-1
  Gain2 : Gain
  Gain3 : Gain  Gain=0
  Gain4 : Gain  Gain=0
  Gain5 : Gain
  Gain6 : Gain  Gain=-1.5
  Gain7 : Gain  Gain=4
  Gain8 : Gain  Gain=0
  Mux3 : Mux
  Repeating Sequence5 : Subsystem  mask(Repeating table){rep_seq_t=[0 21 21 24 24 30 30 34 34 36 36 38 38 40 40 45], rep_seq_y=[0 0 1 1 -1 -1 1 1 -1 -1 1 1 -1 -1 0 0]}
      mask prompts: rep_seq_t "Time values:"; rep_seq_y "Output values:"
      mask help: Output a repeating sequence of numbers specified in a table of time-value pairs. Values of time should be monotonically increasing.
      mask init: same as Vicon_16Aug2012/wang jian gcs/Circle/Repeating Sequence4
      mask Help: Repeats cycle given in table. Time values should be monotonically increasing.
      mask Display: plot( disp_seq_t, disp_seq_y )
  Repeating Sequence6 : Subsystem  mask(Repeating table){rep_seq_t=[0 10 10 12 12 15 15 17 17 18 18 19 19 20 20 45], rep_seq_y=[0 0 -1 -1 1 1 -1 -1 1 1 -1 -1 1 1 0 0]}
      mask prompts: rep_seq_t "Time values:"; rep_seq_y "Output values:"
      mask help: Output a repeating sequence of numbers specified in a table of time-value pairs. Values of time should be monotonically increasing.
      mask init: same as Vicon_16Aug2012/wang jian gcs/Circle/Repeating Sequence4
      mask Help: Repeats cycle given in table. Time values should be monotonically increasing.
      mask Display: plot( disp_seq_t, disp_seq_y )
  Repeating Sequence7 : Subsystem  mask(Repeating table){rep_seq_t=[0 2 2 5 5 7 7  8 8 9 9 10 10 45], rep_seq_y=[0.5 0.5 1.5 1.5 0.5 0.5 1.5 1.5 0.5 0.5 1.5 1.5 1 1]*-1}
      mask prompts: rep_seq_t "Time values:"; rep_seq_y "Output values:"
      mask help: Output a repeating sequence of numbers specified in a table of time-value pairs. Values of time should be monotonically increasing.
      mask init: same as Vicon_16Aug2012/wang jian gcs/Circle/Repeating Sequence4
      mask Help: Repeats cycle given in table. Time values should be monotonically increasing.
      mask Display: plot( disp_seq_t, disp_seq_y )
  Repeating Sequence8 : Subsystem  mask(Repeating table){rep_seq_t=[0 44 44 45 45], rep_seq_y=[0 0 -1 -1 0]*pi/4}
      mask prompts: rep_seq_t "Time values:"; rep_seq_y "Output values:"
      mask help: Output a repeating sequence of numbers specified in a table of time-value pairs. Values of time should be monotonically increasing.
      mask init: same as Vicon_16Aug2012/wang jian gcs/Circle/Repeating Sequence4
      mask Help: Repeats cycle given in table. Time values should be monotonically increasing.
      mask Display: plot( disp_seq_t, disp_seq_y )
  POS : Outport  OutputWhenDisabled=reset  InitialOutput=[0 0 0.2 0]
  wires:
  Gain8/1 -> Mux3/4
  Repeating Sequence7/1(Out1) -> Gain5/1
  Repeating Sequence6/1(Out1) -> Gain6/1
  Repeating Sequence5/1(Out1) -> Gain7/1
  Repeating Sequence8/1(Out1) -> ?
  Gain4/1 -> Mux3/2
  Gain3/1 -> Mux3/1
  Mux3/1 -> Gain2/1
  Discrete-Time Integrator4/1 -> Gain4/1, Gain3/1, Gain8/1, Gain1/1
  Constant1/1 -> Discrete-Time Integrator4/1
  Gain2/1 -> POS/1
  Gain1/1 -> Mux3/3

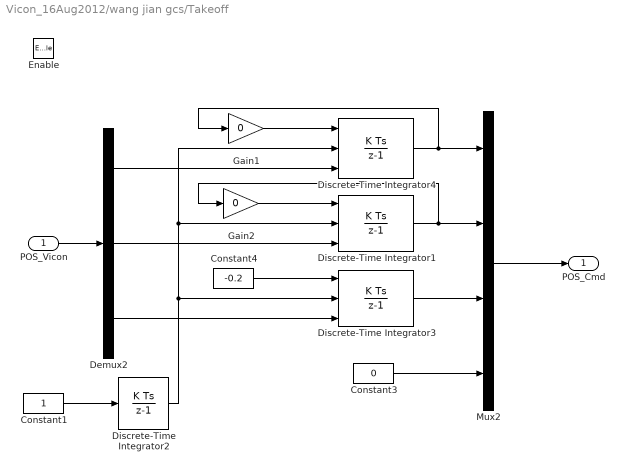
== system Vicon_16Aug2012/wang jian gcs/Takeoff ==
  POS_Vicon : Inport
  Enable : EnablePort  StatesWhenEnabling=reset
  Constant1 : Constant  OutDataTypeStr=double
  Constant3 : Constant  Value=0  OutDataTypeStr=double
  Constant4 : Constant  Value=-0.2  OutDataTypeStr=double
  Demux2 : Demux  Outputs=3
  Discrete-Time Integrator1 : DiscreteIntegrator  ExternalReset=rising  InitialConditionSource=external  SampleTime=sample_time  LimitOutput=on  UpperSaturationLimit=3  LowerSaturationLimit=-3  ICPrevOutput=DiscIntNeverNeededParam  ICPrevScaledInput=DiscIntNeverNeededParam
  Discrete-Time Integrator2 : DiscreteIntegrator  SampleTime=-1  ICPrevOutput=DiscIntNeverNeededParam  ICPrevScaledInput=DiscIntNeverNeededParam
  Discrete-Time Integrator3 : DiscreteIntegrator  ExternalReset=rising  InitialConditionSource=external  SampleTime=sample_time  LimitOutput=on  UpperSaturationLimit=0.2  LowerSaturationLimit=-0.8  ICPrevOutput=DiscIntNeverNeededParam  ICPrevScaledInput=DiscIntNeverNeededParam
  Discrete-Time Integrator4 : DiscreteIntegrator  ExternalReset=rising  InitialConditionSource=external  SampleTime=sample_time  LimitOutput=on  UpperSaturationLimit=1  LowerSaturationLimit=-1  ICPrevOutput=DiscIntNeverNeededParam  ICPrevScaledInput=DiscIntNeverNeededParam
  Gain1 : Gain  Gain=0
  Gain2 : Gain  Gain=0
  Mux2 : Mux
  POS_Cmd : Outport  OutputWhenDisabled=reset  InitialOutput=[0 0 -0.8 0]
  wires:
  Discrete-Time Integrator1/1 -> Mux2/2, Gain2/1
  Gain2/1 -> Discrete-Time Integrator1/1
  Demux2/3 -> Discrete-Time Integrator3/3
  Demux2/2 -> Discrete-Time Integrator1/3
  Demux2/1 -> Discrete-Time Integrator4/3
  POS_Vicon/1 -> Demux2/1
  Discrete-Time Integrator4/1 -> Mux2/1, Gain1/1
  Constant4/1 -> Discrete-Time Integrator3/1
  Discrete-Time Integrator2/1 -> Discrete-Time Integrator3/2, Discrete-Time Integrator1/2, Discrete-Time Integrator4/2
  Constant1/1 -> Discrete-Time Integrator2/1
  Constant3/1 -> Mux2/4
  Gain1/1 -> Discrete-Time Integrator4/1
  Mux2/1 -> POS_Cmd/1
  Discrete-Time Integrator3/1 -> Mux2/3

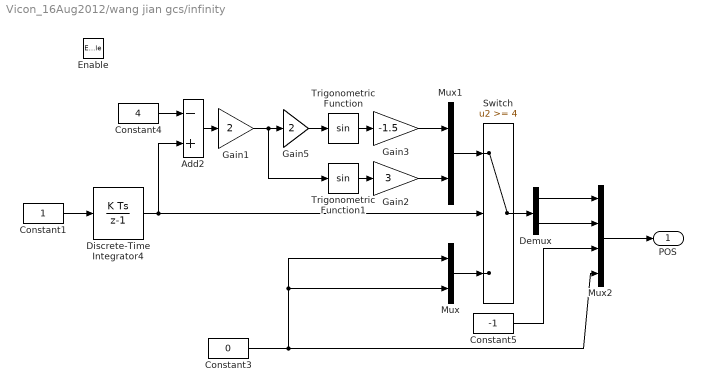
== system Vicon_16Aug2012/wang jian gcs/infinity ==
  Enable : EnablePort  StatesWhenEnabling=reset
  Add2 : Sum  Inputs=-+
  Constant1 : Constant  OutDataTypeStr=double
  Constant3 : Constant  Value=0  OutDataTypeStr=double
  Constant4 : Constant  Value=4  OutDataTypeStr=double
  Constant5 : Constant  Value=-1  OutDataTypeStr=double
  Demux : Demux  Outputs=2
  Discrete-Time Integrator4 : DiscreteIntegrator  SampleTime=-1  ICPrevOutput=DiscIntNeverNeededParam  ICPrevScaledInput=DiscIntNeverNeededParam
  Gain1 : Gain  Gain=2
  Gain2 : Gain  Gain=3
  Gain3 : Gain  Gain=-1.5
  Gain5 : Gain  Gain=2
  Mux : Mux  Inputs=2
  Mux1 : Mux  Inputs=2
  Mux2 : Mux
  Switch : Switch  Threshold=4
  Trigonometric Function : Trigonometry
  Trigonometric Function1 : Trigonometry
  POS : Outport  OutputWhenDisabled=reset  InitialOutput=[0 0 -0.8 0]
  wires:
  Gain5/1 -> Trigonometric Function/1
  Constant5/1 -> Mux2/3
  Constant1/1 -> Discrete-Time Integrator4/1
  Discrete-Time Integrator4/1 -> Switch/2, Add2/2
  Mux/1 -> Switch/3
  Mux1/1 -> Switch/1
  Trigonometric Function/1 -> Gain3/1
  Trigonometric Function1/1 -> Gain2/1
  Mux2/1 -> POS/1
  Switch/1 -> Demux/1
  Demux/1 -> Mux2/1
  Demux/2 -> Mux2/2
  Constant3/1 -> Mux/2, Mux/1, Mux2/4
  Gain3/1 -> Mux1/1
  Gain2/1 -> Mux1/2
  Gain1/1 -> Trigonometric Function1/1, Gain5/1
  Constant4/1 -> Add2/1
  Add2/1 -> Gain1/1

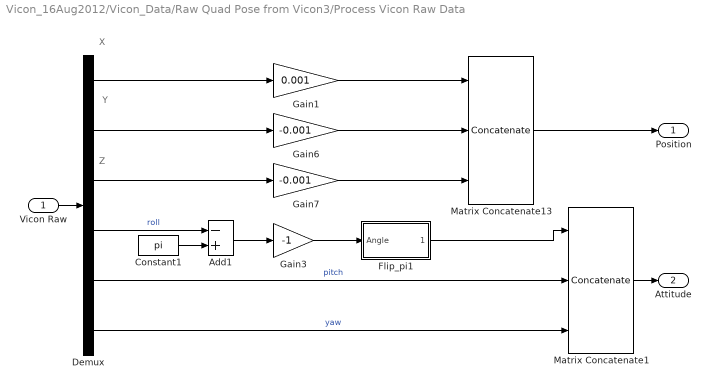
== system Vicon_16Aug2012/Vicon_Data/Raw Quad Pose from Vicon3/Process Vicon Raw Data ==
  note: X
  note: Y
  note: Z
  Vicon Raw : Inport
  Add1 : Sum  Inputs=-+
  Constant1 : Constant  Value=pi  OutDataTypeStr=double
  Demux : Demux  Outputs=6
  Flip_pi1 : Subsystem
      mask Type: Flip -pi to pi
      mask Description: Flips the inputs into the range -pi to pi
      mask Help: Flips the inputs into the range -pi to pi
      mask Display: disp('Flip_pi')
  Gain1 : Gain  Gain=0.001
  Gain3 : Gain  Gain=-1
  Gain6 : Gain  Gain=-0.001
  Gain7 : Gain  Gain=-0.001
  Matrix Concatenate1 : Concatenate  NumInputs=3  Mode=Multidimensional array
  Matrix Concatenate13 : Concatenate  NumInputs=3  Mode=Multidimensional array
  Position : Outport
  Attitude : Outport  Port=2
  wires:
  Constant1/1 -> Add1/2
  Demux/6 -> Matrix Concatenate1/3  "yaw"
  Gain1/1 -> Matrix Concatenate13/1
  Demux/1 -> Gain1/1
  Demux/2 -> Gain6/1
  Demux/3 -> Gain7/1
  Demux/4 -> Add1/1  "roll"
  Gain6/1 -> Matrix Concatenate13/2
  Gain7/1 -> Matrix Concatenate13/3
  Add1/1 -> Gain3/1
  Gain3/1 -> Flip_pi1/1(Angle)
  Demux/5 -> Matrix Concatenate1/2  "pitch"
  Flip_pi1/1(Angle_Flip) -> Matrix Concatenate1/1
  Matrix Concatenate13/1 -> Position/1
  Vicon Raw/1 -> Demux/1
  Matrix Concatenate1/1 -> Attitude/1

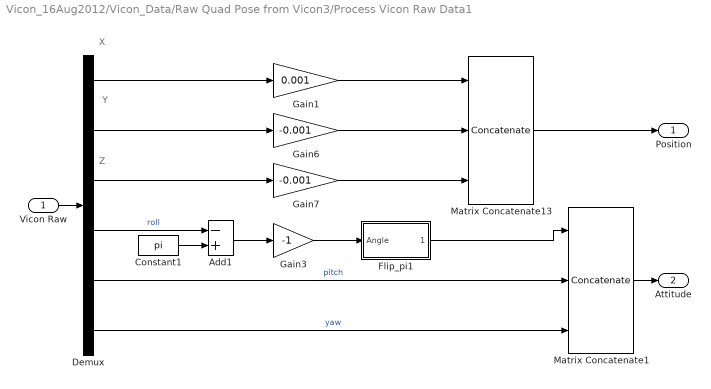
== system Vicon_16Aug2012/Vicon_Data/Raw Quad Pose from Vicon3/Process Vicon Raw Data1 ==
  note: Z
  note: Y
  note: X
  Vicon Raw : Inport
  Add1 : Sum  Inputs=-+
  Constant1 : Constant  Value=pi  OutDataTypeStr=double
  Demux : Demux  Outputs=6
  Flip_pi1 : Subsystem
      mask Type: Flip -pi to pi
      mask Description: Flips the inputs into the range -pi to pi
      mask Help: Flips the inputs into the range -pi to pi
      mask Display: disp('Flip_pi')
  Gain1 : Gain  Gain=0.001
  Gain3 : Gain  Gain=-1
  Gain6 : Gain  Gain=-0.001
  Gain7 : Gain  Gain=-0.001
  Matrix Concatenate1 : Concatenate  NumInputs=3  Mode=Multidimensional array
  Matrix Concatenate13 : Concatenate  NumInputs=3  Mode=Multidimensional array
  Position : Outport
  Attitude : Outport  Port=2
  wires:
  Matrix Concatenate1/1 -> Attitude/1
  Vicon Raw/1 -> Demux/1
  Matrix Concatenate13/1 -> Position/1
  Flip_pi1/1(Angle_Flip) -> Matrix Concatenate1/1
  Demux/5 -> Matrix Concatenate1/2  "pitch"
  Gain3/1 -> Flip_pi1/1(Angle)
  Add1/1 -> Gain3/1
  Gain7/1 -> Matrix Concatenate13/3
  Gain6/1 -> Matrix Concatenate13/2
  Demux/4 -> Add1/1  "roll"
  Demux/3 -> Gain7/1
  Demux/2 -> Gain6/1
  Demux/1 -> Gain1/1
  Gain1/1 -> Matrix Concatenate13/1
  Demux/6 -> Matrix Concatenate1/3  "yaw"
  Constant1/1 -> Add1/2

== system Vicon_16Aug2012/Vicon_Data/Raw Quad Pose from Vicon3/Process Vicon Raw Data2 ==
  note: X
  note: Y
  note: Z
  Vicon Raw : Inport
  Add1 : Sum  Inputs=-+
  Constant1 : Constant  Value=pi  OutDataTypeStr=double
  Demux : Demux  Outputs=6
  Flip_pi1 : Subsystem
      mask Type: Flip -pi to pi
      mask Description: Flips the inputs into the range -pi to pi
      mask Help: Flips the inputs into the range -pi to pi
      mask Display: disp('Flip_pi')
  Gain1 : Gain  Gain=0.001
  Gain3 : Gain  Gain=-1
  Gain6 : Gain  Gain=-0.001
  Gain7 : Gain  Gain=-0.001
  Matrix Concatenate1 : Concatenate  NumInputs=3  Mode=Multidimensional array
  Matrix Concatenate13 : Concatenate  NumInputs=3  Mode=Multidimensional array
  Position : Outport
  Attitude : Outport  Port=2
  wires:
  Constant1/1 -> Add1/2
  Demux/6 -> Matrix Concatenate1/3  "yaw"
  Gain1/1 -> Matrix Concatenate13/1
  Demux/1 -> Gain1/1
  Demux/2 -> Gain6/1
  Demux/3 -> Gain7/1
  Demux/4 -> Add1/1  "roll"
  Gain6/1 -> Matrix Concatenate13/2
  Gain7/1 -> Matrix Concatenate13/3
  Add1/1 -> Gain3/1
  Gain3/1 -> Flip_pi1/1(Angle)
  Demux/5 -> Matrix Concatenate1/2  "pitch"
  Flip_pi1/1(Angle_Flip) -> Matrix Concatenate1/1
  Matrix Concatenate13/1 -> Position/1
  Vicon Raw/1 -> Demux/1
  Matrix Concatenate1/1 -> Attitude/1

== system Vicon_16Aug2012/wang jian gcs/Circle/Repeating Sequence4 ==
  Time_Enabled : Inport
  Constant : Constant  DisableCoverage=on  Value=period
  Look-Up Table1 : Lookup  DisableCoverage=on  InputValues=rep_seq_t - min(rep_seq_t)  Table=rep_seq_y  SaturateOnIntegerOverflow=on
  Math Function : Math  DisableCoverage=on  Operator=rem  SaturateOnIntegerOverflow=on
  Output : SignalConversion  ConversionOutput=Contiguous copy
  Sum : Sum  DisableCoverage=on  Inputs=+-  SaturateOnIntegerOverflow=on  InputSameDT=on  OutDataTypeStr=Inherit: Same as first input
  startTime : S-Function  DisableCoverage=on  FunctionName=sfun_tstart  EnableBusSupport=off
  Out1 : Outport
  wires:
  Constant/1 -> Math Function/2
  Output/1 -> Out1/1
  Look-Up Table1/1 -> Output/1
  startTime/1 -> Sum/2
  Time_Enabled/1 -> Sum/1
  Sum/1 -> Math Function/1
  Math Function/1 -> Look-Up Table1/1

== system Vicon_16Aug2012/wang jian gcs/RC_Control/PT2 ==
  u : Inport
  u1 : Inport  Port=2
  Constant : Constant  Value=T
  Discrete-Time Integrator : DiscreteIntegrator  ExternalReset=rising  InitialConditionSource=external  SampleTime=sample_time  ICPrevOutput=DiscIntNeverNeededParam  ICPrevScaledInput=DiscIntNeverNeededParam
  Divide : Product  Inputs=*/
  Step : Step  Time=0.2
  Sum : Sum  Inputs=|+-
  y : Outport
  wires:
  u/1 -> Sum/1
  Sum/1 -> Divide/1
  Step/1 -> Discrete-Time Integrator/2
  Discrete-Time Integrator/1 -> Sum/2, y/1
  Divide/1 -> Discrete-Time Integrator/1
  Constant/1 -> Divide/2
  u1/1 -> Discrete-Time Integrator/3

== system Vicon_16Aug2012/wang jian gcs/Steps/Repeating Sequence5 ==
  Time_Enabled : Inport
  Constant : Constant  DisableCoverage=on  Value=period
  Look-Up Table1 : Lookup  DisableCoverage=on  InputValues=rep_seq_t - min(rep_seq_t)  Table=rep_seq_y  SaturateOnIntegerOverflow=on
  Math Function : Math  DisableCoverage=on  Operator=rem  SaturateOnIntegerOverflow=on
  Output : SignalConversion  ConversionOutput=Contiguous copy
  Sum : Sum  DisableCoverage=on  Inputs=+-  SaturateOnIntegerOverflow=on  InputSameDT=on  OutDataTypeStr=Inherit: Same as first input
  startTime : S-Function  DisableCoverage=on  FunctionName=sfun_tstart  EnableBusSupport=off
  Out1 : Outport
  wires:
  Constant/1 -> Math Function/2
  Output/1 -> Out1/1
  Look-Up Table1/1 -> Output/1
  startTime/1 -> Sum/2
  Time_Enabled/1 -> Sum/1
  Sum/1 -> Math Function/1
  Math Function/1 -> Look-Up Table1/1

== system Vicon_16Aug2012/wang jian gcs/Steps/Repeating Sequence6 ==
  Time_Enabled : Inport
  Constant : Constant  DisableCoverage=on  Value=period
  Look-Up Table1 : Lookup  DisableCoverage=on  InputValues=rep_seq_t - min(rep_seq_t)  Table=rep_seq_y  SaturateOnIntegerOverflow=on
  Math Function : Math  DisableCoverage=on  Operator=rem  SaturateOnIntegerOverflow=on
  Output : SignalConversion  ConversionOutput=Contiguous copy
  Sum : Sum  DisableCoverage=on  Inputs=+-  SaturateOnIntegerOverflow=on  InputSameDT=on  OutDataTypeStr=Inherit: Same as first input
  startTime : S-Function  DisableCoverage=on  FunctionName=sfun_tstart  EnableBusSupport=off
  Out1 : Outport
  wires:
  Math Function/1 -> Look-Up Table1/1
  Sum/1 -> Math Function/1
  Time_Enabled/1 -> Sum/1
  startTime/1 -> Sum/2
  Look-Up Table1/1 -> Output/1
  Output/1 -> Out1/1
  Constant/1 -> Math Function/2

== system Vicon_16Aug2012/wang jian gcs/Steps/Repeating Sequence7 ==
  Time_Enabled : Inport
  Constant : Constant  DisableCoverage=on  Value=period
  Look-Up Table1 : Lookup  DisableCoverage=on  InputValues=rep_seq_t - min(rep_seq_t)  Table=rep_seq_y  SaturateOnIntegerOverflow=on
  Math Function : Math  DisableCoverage=on  Operator=rem  SaturateOnIntegerOverflow=on
  Output : SignalConversion  ConversionOutput=Contiguous copy
  Sum : Sum  DisableCoverage=on  Inputs=+-  SaturateOnIntegerOverflow=on  InputSameDT=on  OutDataTypeStr=Inherit: Same as first input
  startTime : S-Function  DisableCoverage=on  FunctionName=sfun_tstart  EnableBusSupport=off
  Out1 : Outport
  wires:
  Math Function/1 -> Look-Up Table1/1
  Sum/1 -> Math Function/1
  Time_Enabled/1 -> Sum/1
  startTime/1 -> Sum/2
  Look-Up Table1/1 -> Output/1
  Output/1 -> Out1/1
  Constant/1 -> Math Function/2

== system Vicon_16Aug2012/wang jian gcs/Steps/Repeating Sequence8 ==
  Time_Enabled : Inport
  Constant : Constant  DisableCoverage=on  Value=period
  Look-Up Table1 : Lookup  DisableCoverage=on  InputValues=rep_seq_t - min(rep_seq_t)  Table=rep_seq_y  SaturateOnIntegerOverflow=on
  Math Function : Math  DisableCoverage=on  Operator=rem  SaturateOnIntegerOverflow=on
  Output : SignalConversion  ConversionOutput=Contiguous copy
  Sum : Sum  DisableCoverage=on  Inputs=+-  SaturateOnIntegerOverflow=on  InputSameDT=on  OutDataTypeStr=Inherit: Same as first input
  startTime : S-Function  DisableCoverage=on  FunctionName=sfun_tstart  EnableBusSupport=off
  Out1 : Outport
  wires:
  Constant/1 -> Math Function/2
  Output/1 -> Out1/1
  Look-Up Table1/1 -> Output/1
  startTime/1 -> Sum/2
  Time_Enabled/1 -> Sum/1
  Sum/1 -> Math Function/1
  Math Function/1 -> Look-Up Table1/1

== system Vicon_16Aug2012/Vicon_Data/Raw Quad Pose from Vicon3/Process Vicon Raw Data/Flip_pi1 ==
  Angle : Inport
  Add : Sum  Inputs=-+
  Compare To Constant1 : simulink/Logic and Bit Operations/Compare To Constant  SystemSampleTime=-1  relop=>  const=pi  LogicOutDataTypeMode=uint8  ZeroCross=off
  Constant : Constant  Value=2*pi
  Data Type Duplicate : DataTypeDuplicate
  Flip_0_to_2pi : Subsystem
      mask Type: Flip zero to 2pi
      mask Description: Flips the inputs into the range zero to +2pi
      mask Help: Flips the inputs into the range zero to +2pi
      mask Display: disp('Flip_0_2pi')
  Switch : Switch  Criteria=u2 ~= 0
  Angle_Flip : Outport
  wires:
  Switch/1 -> Data Type Duplicate/1, Angle_Flip/1
  Add/1 -> Switch/1
  Constant/1 -> Add/1
  Compare To Constant1/1 -> Switch/2
  Flip_0_to_2pi/1(Angle_Flip) -> Add/2, Compare To Constant1/1, Switch/3
  Angle/1 -> Data Type Duplicate/2, Flip_0_to_2pi/1(Angle)

== system Vicon_16Aug2012/Vicon_Data/Raw Quad Pose from Vicon3/Process Vicon Raw Data1/Flip_pi1 ==
  Angle : Inport
  Add : Sum  Inputs=-+
  Compare To Constant1 : simulink/Logic and Bit Operations/Compare To Constant  SystemSampleTime=-1  relop=>  const=pi  LogicOutDataTypeMode=uint8  ZeroCross=off
  Constant : Constant  Value=2*pi
  Data Type Duplicate : DataTypeDuplicate
  Flip_0_to_2pi : Subsystem
      mask Type: Flip zero to 2pi
      mask Description: Flips the inputs into the range zero to +2pi
      mask Help: Flips the inputs into the range zero to +2pi
      mask Display: disp('Flip_0_2pi')
  Switch : Switch  Criteria=u2 ~= 0
  Angle_Flip : Outport
  wires:
  Angle/1 -> Flip_0_to_2pi/1(Angle), Data Type Duplicate/2
  Flip_0_to_2pi/1(Angle_Flip) -> Switch/3, Compare To Constant1/1, Add/2
  Compare To Constant1/1 -> Switch/2
  Constant/1 -> Add/1
  Add/1 -> Switch/1
  Switch/1 -> Angle_Flip/1, Data Type Duplicate/1

== system Vicon_16Aug2012/Vicon_Data/Raw Quad Pose from Vicon3/Process Vicon Raw Data2/Flip_pi1 ==
  Angle : Inport
  Add : Sum  Inputs=-+
  Compare To Constant1 : simulink/Logic and Bit Operations/Compare To Constant  SystemSampleTime=-1  relop=>  const=pi  LogicOutDataTypeMode=uint8  ZeroCross=off
  Constant : Constant  Value=2*pi
  Data Type Duplicate : DataTypeDuplicate
  Flip_0_to_2pi : Subsystem
      mask Type: Flip zero to 2pi
      mask Description: Flips the inputs into the range zero to +2pi
      mask Help: Flips the inputs into the range zero to +2pi
      mask Display: disp('Flip_0_2pi')
  Switch : Switch  Criteria=u2 ~= 0
  Angle_Flip : Outport
  wires:
  Switch/1 -> Data Type Duplicate/1, Angle_Flip/1
  Add/1 -> Switch/1
  Constant/1 -> Add/1
  Compare To Constant1/1 -> Switch/2
  Flip_0_to_2pi/1(Angle_Flip) -> Add/2, Compare To Constant1/1, Switch/3
  Angle/1 -> Data Type Duplicate/2, Flip_0_to_2pi/1(Angle)

== system Vicon_16Aug2012/Vicon_Data/Raw Quad Pose from Vicon3/Process Vicon Raw Data/Flip_pi1/Flip_0_to_2pi ==
  Angle : Inport
  Add : Sum
  Compare To Constant1 : simulink/Logic and Bit Operations/Compare To Constant  SystemSampleTime=-1  relop=<  const=0  LogicOutDataTypeMode=uint8  ZeroCross=off
  Constant : Constant  Value=2*pi
  Data Type Duplicate : DataTypeDuplicate
  Flip_2pi : Subsystem
      mask Type: Flip -2pi to 2pi
      mask Description: Flips the inputs into the range -2pi to +2pi
      mask Help: Flips the inputs into the range -2pi to +2pi
      mask Display: disp('Flip_2pi')
  Switch : Switch  Criteria=u2 ~= 0
  Angle_Flip : Outport
  wires:
  Switch/1 -> Data Type Duplicate/1, Angle_Flip/1
  Angle/1 -> Data Type Duplicate/2, Flip_2pi/1(Angle)
  Add/1 -> Switch/1
  Constant/1 -> Add/1
  Compare To Constant1/1 -> Switch/2
  Flip_2pi/1(Angle_Flip) -> Switch/3, Add/2, Compare To Constant1/1

== system Vicon_16Aug2012/Vicon_Data/Raw Quad Pose from Vicon3/Process Vicon Raw Data1/Flip_pi1/Flip_0_to_2pi ==
  Angle : Inport
  Add : Sum
  Compare To Constant1 : simulink/Logic and Bit Operations/Compare To Constant  SystemSampleTime=-1  relop=<  const=0  LogicOutDataTypeMode=uint8  ZeroCross=off
  Constant : Constant  Value=2*pi
  Data Type Duplicate : DataTypeDuplicate
  Flip_2pi : Subsystem
      mask Type: Flip -2pi to 2pi
      mask Description: Flips the inputs into the range -2pi to +2pi
      mask Help: Flips the inputs into the range -2pi to +2pi
      mask Display: disp('Flip_2pi')
  Switch : Switch  Criteria=u2 ~= 0
  Angle_Flip : Outport
  wires:
  Flip_2pi/1(Angle_Flip) -> Compare To Constant1/1, Add/2, Switch/3
  Compare To Constant1/1 -> Switch/2
  Constant/1 -> Add/1
  Add/1 -> Switch/1
  Angle/1 -> Flip_2pi/1(Angle), Data Type Duplicate/2
  Switch/1 -> Angle_Flip/1, Data Type Duplicate/1
